simulink model "characterization"  (R2024a)
settings: Solver=FixedStepDiscrete  StartTime=0.0  StopTime=500  FixedStep=0.005  RelTol=1e-3
undefined symbols (not defined in the file): V_final, V_initial
libraries: simulink x1
settings Model: SimulationMode=external  Creator=Bocchio  LastModifiedBy=Bocchio
settings DataIOCC: SaveFormat=Array  SaveOutput=off  SaveTime=off  ReturnWorkspaceOutputs=off
settings HardwareCC: ProdBitPerPointer=32  ProdBitPerSizeT=32  ProdBitPerPtrDiffT=32  ProdLargestAtomicFloat=None  ProdIntDivRoundTo=Undefined  ProdEndianess=Unspecified  ProdWordSize=32  ProdHWDeviceType=Custom Processor->Custom Processor
settings ModelReferenceCC: EnableRefExpFcnMdlSchedulingChecks=on  PropagateSignalLabelsOutOfModel=off
settings SFSimCC: CustomCodeUndefinedFunction=UseInterfaceOnly
settings RTWCC: Description=MLS2EM-RTDAC/USB2 (Visual C/C++)  SystemTargetFile=mls2em_rtcon_usb2.tlc  TemplateMakefile=MLS2EM_RTCON_VC_USB2_x64.tmf
settings CodeAppCC: StateflowObjectComments=on
settings STFCustomTargetCC: ModelReferenceCompliant=off  CombineOutputUpdateFcns=on  MatFileLogging=on  GRTInterface=off  UseToolchainInfoCompliant=off  SystemTargetFile=mls2em_rtcon_usb2.tlc
settings GRTTargetCC: ModelReferenceCompliant=off  ParMdlRefBuildCompliant=off  CompOptLevelCompliant=off  ConcurrentExecutionCompliant=off  CPPClassGenCompliant=off  UseToolchainInfoCompliant=off  ExtMode=on  ExtModeMexFile=rtcon_ext_comm

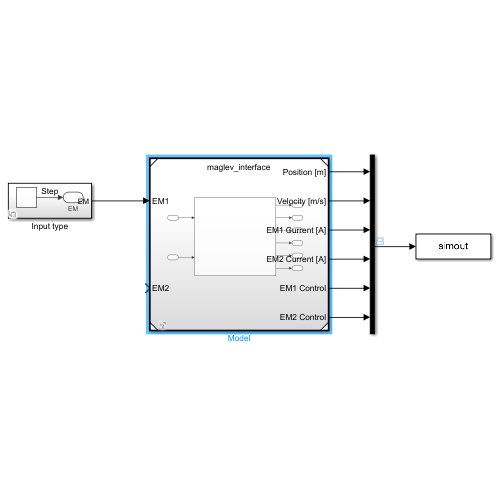
[thumbnail: Simulink's stored preview of the top-level diagram]
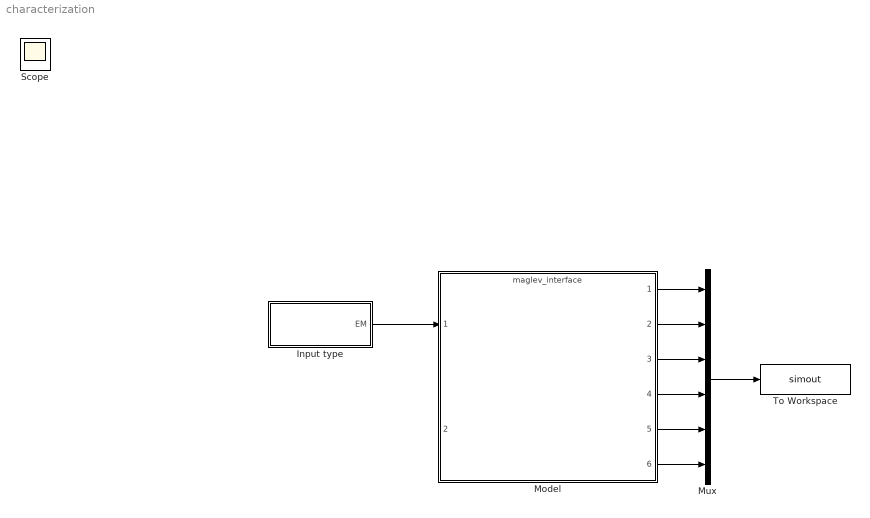
== system characterization ==
  Input type : Subsystem  Variant=on
  Model : ModelReference  ModelNameDialog=maglev_interface.slx  SimulationMode=Normal  ModelReferenceVersion=9.1
  Mux : Mux  Inputs=6
  To Workspace : ToWorkspace  VariableName=simout  SaveFormat=Timeseries  SampleTime=-1
  Scope : Scope
  wires:
  Model/1 -> Mux/1
  Model/2 -> Mux/2
  Model/3 -> Mux/3
  Model/4 -> Mux/4
  Model/5 -> Mux/5
  Model/6 -> Mux/6
  Mux/1 -> To Workspace/1
  Input type/1(EM) -> Model/1

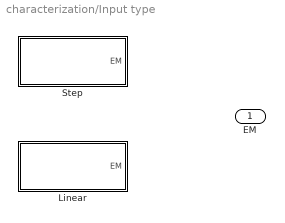
== system characterization/Input type ==
  Linear : Subsystem  VariantControl=false
  Step : Subsystem  VariantControl=true
  EM : Outport

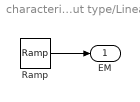
== system characterization/Input type/Linear ==
  Ramp : simulink/Sources/Ramp  slope=(V_final - V_initial) / 10  start=t_start  InitialOutput=V_initial
  EM : Outport
  wires:
  Ramp/1 -> EM/1

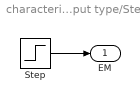
== system characterization/Input type/Step ==
  Step : Step  SampleTime=0
  EM : Outport
  wires:
  Step/1 -> EM/1
